simulink model "gm_uc3_preparation1_2017"  (R2018a)
settings: Solver=FixedStepDiscrete  StartTime=0.0  StopTime=0.6  FixedStep=2e-5  RelTol=1e-3  EnableMultiTasking=on
libraries: hdlsllib x6, simulink x3
(part 2 of 2)

== matlab function gm_uc3_preparation1_2017/CandHDL_c/cgenerate/Subsystem/RT_CPU ==
  data: A input [0..1]; f input; cc output; strobe output; mode input [0..2]; din input [0..100]; n input [0..3]; b output
function [cc,strobe,b]  = fcn(A,f,mode,din,n)
%% RT CPU
%   This Embedded Matlab function calculates the polynomial coefficients
%       and breaks points according to the external user settings. 
%       Three different waveforms can be selected with "mode"
%               0: Sine
%               1: Rectangular (not implemented yet)
%               2: Triangular  (not implemented yet)
%
%       
%    Author: R. Estrada, FH JOANNEUM, 2018
%
%%
    % Declaration of global variables
    persistent cc0 b0 i0 ;
    d=din
    d_sep=(din*1.28)
    % This is executed only once during Initialization
    if isempty(cc0)    
        cc0 =  single(zeros(129,3));  %    zeros(101,3);
        b0  = single(zeros(1,129)); %zeros(1,101);
        nb = single(128);
        n = single(2);
        
        cc =  single(zeros(129,3));
        b  = single(zeros(1,129));
        i0=single(0);
         
    end
    strobe=single(0);
    
    % Calculation is done only once
    %  Note: An external signal together with an OR condition can be added
    %        for recalculating the coefficients and break points on demand
    if i0<single(1)        
        i0=single(1);

         cc = single(zeros(129,3));   
         b  = single(zeros(1,129));
         nb = single(128);
         tf = single(1/f);
         
         strobe=single(1);
         assert(nb<=256);

         %d=single(1);
         
         
        switch mode
            case 0 % Sine wave
               % nb = 100;        % Number of break points
                %n  = 2;         % Polynomial order
                %y  = A*sin(2*pi*f.*linspace(0,1/f,nb+1));        
                y  = single(A*sin(2*pi*f.*linspace(0,1/f,129))); 
                
            case 1 %Rectangle wave 
               
                %assert((A>0)&&(A<=1));
               % assert(nb<=256);
                i=1;
                y=single(zeros(1,129));
             
               for j=0:tf/(128):tf
                  if  j<=tf*d
                   
                        y(i)=single(A);
                    else
                        y(i)=-single(A);
                  end
                    i=i+1;
                end
                
            case 2 %triangle wave
                
                i=1;
                  y=single(zeros(1,129));
                  for j=0:tf/(128):tf
                      if i==1
                            y(i)=single(A);
                      else
                          if j<=tf*d
                              y(i)=single(y(i-1)+2*(A/128)/(d));
                          else
                              y(i)=single(y(i-1)-2*(A/128)/(1-d));
                          end
                      end
                      i=i+1;
                  end 
            case 3
                 
                %assert((A>0)&&(A<=1));
               % assert(nb<=256);
                      y=single(zeros(1,129));
             
               for j=1:128
                  if  j<=d_sep
                   
                        y(j)=single(A);
                    else
                        y(j)=-single(A);
                  end
                    y(j+1)=A;
                    
               end
        
            case 4
                y=single(zeros(1,129));
                    for i=1:128
                        if i<=d_sep
                            y(i)=single(A-(A/d_sep));
                        else
                            y(i)=single(-1*A+(A/(128-d_sep-i)));
                        end
                         
                    end
                     y(i+1)=A;
                
              
            otherwise
                nb = single(128);
                n = single(2);
               y=single(zeros(1,129));
        end

        %% Finite difference
        %   Coefficients
        cfd = [  1 0 0 0;...
                -1 1 0 0; ...
                 1 -2 1 0; ...
                -1 3 -3 1];

        % Extend array around the end
        yy = [y y(2:4)];
        
        for j=0:1:nb                        % Sweep of break points
            b(1,j+1)=j*tf/nb;               % Store actual break point
            ys = [yy(j+1) yy(j+2) yy(j+3) yy(j+4)];   % Prepare y vector
            for i=0:1:n       
                dy = cfd(i+1,:) * ys'/(f/nb)^i; % Compute n derivate        
                cc(j+1,i+1)= dy/factorial(i);        
            end                  
        end
        
        % Store values in global variables
        cc0 = cc;  
        b0  = b;
     %   strobe0=strobe;
    else
        % Keep the previous values
        cc = cc0;
        b  = b0;
    
    end %end of main if
    
end % Function
